simulink model "ADS_model_S2019a"  (R2019a)
settings: Solver=FixedStepDiscrete  StartTime=0.0  StopTime=inf  FixedStep=1/100  RelTol=1e-3
libraries: sldrtlib x2
settings Model: Creator=Admin  LastModifiedBy=Martin Dodek
settings DataIOCC: ReturnWorkspaceOutputs=off
settings DebuggingCC: PregeneratedLibrarySubsystemCodeDiagnostic=none  ArithmeticOperatorsInVariantConditions=warning
settings SFSimCC: SimUseLocalCustomCode=off
settings RTWCC: RTWUseLocalCustomCode=off

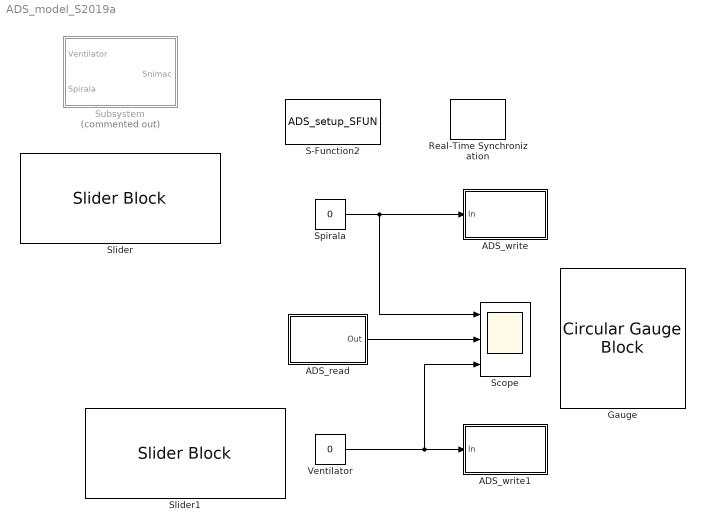
== system ADS_model_S2019a ==
  ADS_read : Subsystem  mask{net_id=[10, 3, 1, 138, 3, 1], var_name='GVL.snimac', var_type=4}
      mask prompts: net_id "net id"; var_name "var name"; var_type "var type"
  ADS_write : Subsystem  mask{net_id=[10, 3, 1, 138, 3, 1], var_name='GVL.spirala', var_type=4}
      mask prompts: net_id "net id"; var_name "var name"; var_type "var type"
  ADS_write1 : Subsystem  mask{net_id=[10, 3, 1, 138, 3, 1], var_name='GVL.ventilator', var_type=4}
      mask prompts: net_id "net id"; var_name "var name"; var_type "var type"
  Gauge : CircularGaugeBlock  ScaleMax=30000
  Real-Time Synchronization : sldrtlib/Real-Time Synchronization  SampleTime=0.01  MaxMissedTicks=100  ShowMissedTicks=off  YieldWhenWaiting=off
  S-Function2 : S-Function  FunctionName=ADS_setup_SFUN  SFunctionDeploymentMode=off  EnableBusSupport=off
  Scope : Scope  NumInputPorts=3
  Slider : SliderBlock  ScaleMax=30000
  Slider1 : SliderBlock  ScaleMax=30000
  Spirala : Constant  Value=0
  Subsystem : Subsystem  Commented=on
  Ventilator : Constant  Value=0
  wires:
  Ventilator/1 -> Scope/3, ADS_write1/1(In)
  Spirala/1 -> Scope/1, ADS_write/1(In)
  ADS_read/1(Out) -> Scope/2

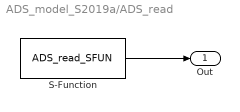
== system ADS_model_S2019a/ADS_read ==
  S-Function : S-Function  FunctionName=ADS_read_SFUN  Parameters=net_id,var_name,var_type  SFunctionDeploymentMode=off  EnableBusSupport=off
  Out : Outport
  wires:
  S-Function/1 -> Out/1

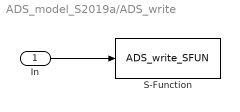
== system ADS_model_S2019a/ADS_write ==
  In : Inport
  S-Function : S-Function  FunctionName=ADS_write_SFUN  Parameters=net_id,var_name,var_type  SFunctionDeploymentMode=off  EnableBusSupport=off
  wires:
  In/1 -> S-Function/1

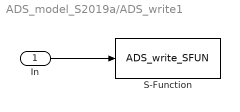
== system ADS_model_S2019a/ADS_write1 ==
  In : Inport
  S-Function : S-Function  FunctionName=ADS_write_SFUN  Parameters=net_id,var_name,var_type  SFunctionDeploymentMode=off  EnableBusSupport=off
  wires:
  In/1 -> S-Function/1

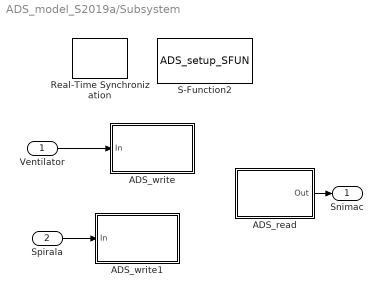
== system ADS_model_S2019a/Subsystem ==
  Ventilator : Inport
  Spirala : Inport  Port=2
  ADS_read : Subsystem  mask{net_id=[10, 3, 1, 138, 3, 1], var_name='GVL.snimac', var_type=4}
      mask prompts: net_id "net id"; var_name "var name"; var_type "var type"
  ADS_write : Subsystem  mask{net_id=[10, 3, 1, 138, 3, 1], var_name='GVL.spirala', var_type=4}
      mask prompts: net_id "net id"; var_name "var name"; var_type "var type"
  ADS_write1 : Subsystem  mask{net_id=[10, 3, 1, 138, 3, 1], var_name='GVL.ventilator', var_type=4}
      mask prompts: net_id "net id"; var_name "var name"; var_type "var type"
  Real-Time Synchronization : sldrtlib/Real-Time Synchronization  SampleTime=0.01  MaxMissedTicks=100  ShowMissedTicks=off  YieldWhenWaiting=off
  S-Function2 : S-Function  FunctionName=ADS_setup_SFUN  SFunctionDeploymentMode=off  EnableBusSupport=off
  Snimac : Outport
  wires:
  ADS_read/1(Out) -> Snimac/1
  Ventilator/1 -> ADS_write/1(In)
  Spirala/1 -> ADS_write1/1(In)

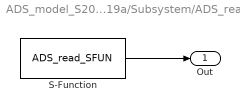
== system ADS_model_S2019a/Subsystem/ADS_read ==
  S-Function : S-Function  FunctionName=ADS_read_SFUN  Parameters=net_id,var_name,var_type  SFunctionDeploymentMode=off  EnableBusSupport=off
  Out : Outport
  wires:
  S-Function/1 -> Out/1

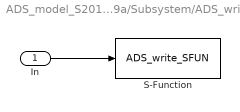
== system ADS_model_S2019a/Subsystem/ADS_write ==
  In : Inport
  S-Function : S-Function  FunctionName=ADS_write_SFUN  Parameters=net_id,var_name,var_type  SFunctionDeploymentMode=off  EnableBusSupport=off
  wires:
  In/1 -> S-Function/1

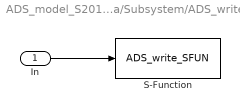
== system ADS_model_S2019a/Subsystem/ADS_write1 ==
  In : Inport
  S-Function : S-Function  FunctionName=ADS_write_SFUN  Parameters=net_id,var_name,var_type  SFunctionDeploymentMode=off  EnableBusSupport=off
  wires:
  In/1 -> S-Function/1
